simulink model "NonlinearBPS"  (R2023b)
settings: Solver=VariableStepAuto  StartTime=0.0  StopTime=10.0  RelTol=1e-3
settings Model: Creator=msdbg  LastModifiedBy=msdbg

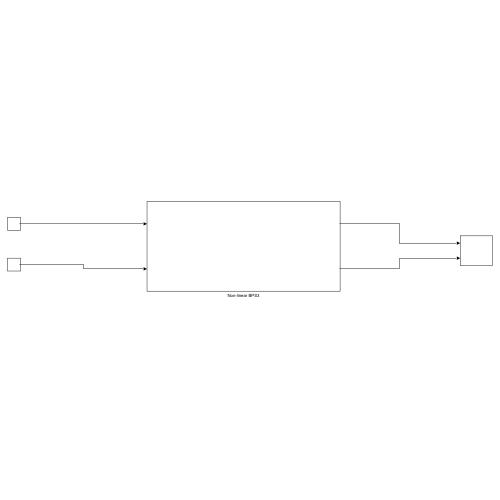
[thumbnail: Simulink's stored preview of the top-level diagram]
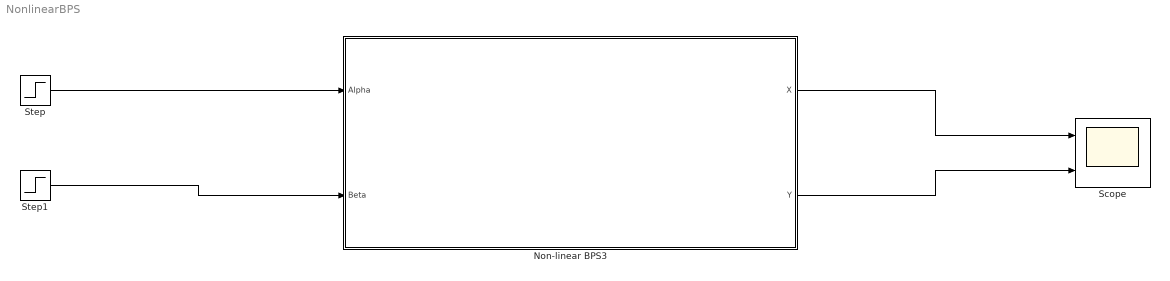
== system NonlinearBPS ==
  Non-linear BPS3 : Subsystem
  Scope : Scope  NumInputPorts=2
  Step : Step  After=3.14/10  SampleTime=0
  Step1 : Step  After=3.14/10  SampleTime=0
  wires:
  Non-linear BPS3/2(Y) -> Scope/2
  Non-linear BPS3/1(X) -> Scope/1
  Step/1 -> Non-linear BPS3/1(Alpha)
  Step1/1 -> Non-linear BPS3/2(Beta)

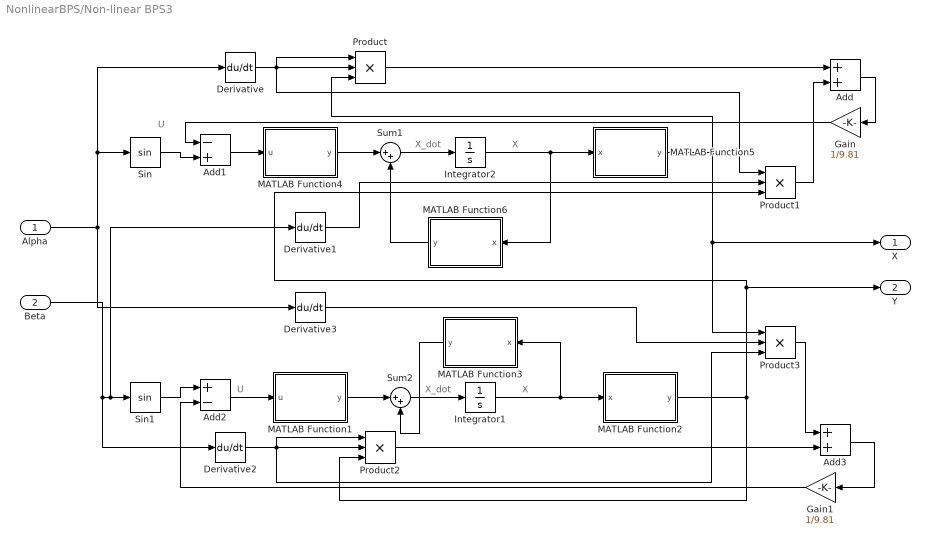
== system NonlinearBPS/Non-linear BPS3 ==
  note: X
  note: U
  note: X_dot
  note: X_dot
  note: U
  note: X
  Alpha : Inport
  Beta : Inport  Port=2
  Add : Sum
  Add1 : Sum  Inputs=-+
  Add2 : Sum  Inputs=+-
  Add3 : Sum
  Derivative{,1..3} (4 alike) : Derivative
  Gain : Gain  Gain=1/9.81
  Gain1 : Gain  Gain=1/9.81
  Integrator1 : Integrator
  Integrator2 : Integrator
  MATLAB Function1 : MATLAB Function  TreatAsAtomicUnit=on
  MATLAB Function2 : MATLAB Function  TreatAsAtomicUnit=on
  MATLAB Function3 : MATLAB Function  TreatAsAtomicUnit=on
  MATLAB Function4 : MATLAB Function  TreatAsAtomicUnit=on
  MATLAB Function5 : MATLAB Function  TreatAsAtomicUnit=on
  MATLAB Function6 : MATLAB Function  TreatAsAtomicUnit=on
  Product{,1..3} (4 alike) : Product  Inputs=3
  Sin : Trigonometry
  Sin1 : Trigonometry
  Sum1 : Sum  Inputs=|++
  Sum2 : Sum  Inputs=|++
  X : Outport  PortDimensions=1
  Y : Outport  Port=2  PortDimensions=1
  wires:
  Beta/1 -> Sin1/1, Derivative1/1, Derivative2/1
  Alpha/1 -> Derivative/1, Sin/1, Derivative3/1
  Integrator2/1 -> MATLAB Function5/1(x), MATLAB Function6/1(x)
  MATLAB Function6/1(y) -> Sum1/2
  Integrator1/1 -> MATLAB Function2/1(x), MATLAB Function3/1(x)
  Product1/1 -> Add/2
  MATLAB Function3/1(y) -> Sum2/2
  MATLAB Function2/1(y) -> Y/1, Product1/3, Product2/3
  Gain1/1 -> Add2/2
  Derivative1/1 -> Product1/2
  MATLAB Function5/1(y) -> X/1, Product3/1, Product/3
  Add3/1 -> Gain1/1
  MATLAB Function4/1(y) -> Sum1/1
  Sin1/1 -> Add2/1
  Sum1/1 -> Integrator2/1
  MATLAB Function1/1(y) -> Sum2/1
  Derivative2/1 -> Product3/3, Product2/2, Product2/1
  Add/1 -> Gain/1
  Derivative/1 -> Product/1, Product1/1, Product/2
  Add2/1 -> MATLAB Function1/1(u)
  Sin/1 -> Add1/2
  Add1/1 -> MATLAB Function4/1(u)
  Derivative3/1 -> Product3/2
  Product2/1 -> Add3/2
  Sum2/1 -> Integrator1/1
  Product/1 -> Add/1
  Product3/1 -> Add3/1
  Gain/1 -> Add1/1

== matlab function NonlinearBPS/Non-linear BPS3/MATLAB Function2 ==
  data: x input; y output
function y = C(x)

y = [1 0]*x;

== matlab function NonlinearBPS/Non-linear BPS3/MATLAB Function3 ==
  data: x input; y output
function y = A(x)

y = [0 1 ; 0 0]*x;

== matlab function NonlinearBPS/Non-linear BPS3/MATLAB Function4 ==
  data: u input; y output
function y = B(u)

y = [0; 5/7*-9.81]*u;

== matlab function NonlinearBPS/Non-linear BPS3/MATLAB Function5 ==
  data: x input; y output
function y = C(x)

y = [1 0]*x;

== matlab function NonlinearBPS/Non-linear BPS3/MATLAB Function6 ==
  data: x input; y output
function y = A(x)

y = [0 1 ; 0 0]*x;

== matlab function NonlinearBPS/Non-linear BPS3/MATLAB Function1 ==
  data: u input; y output
function y = B(u)

y = [0; 5/7*-9.81]*u;
